simulink model "ep_10_26"  (R2023b)
settings: Solver=VariableStepAuto  StartTime=0.0  StopTime=10.0  MaxStep=0.01  RelTol=1e-3
settings Model: Creator=86186  LastModifiedBy=86186

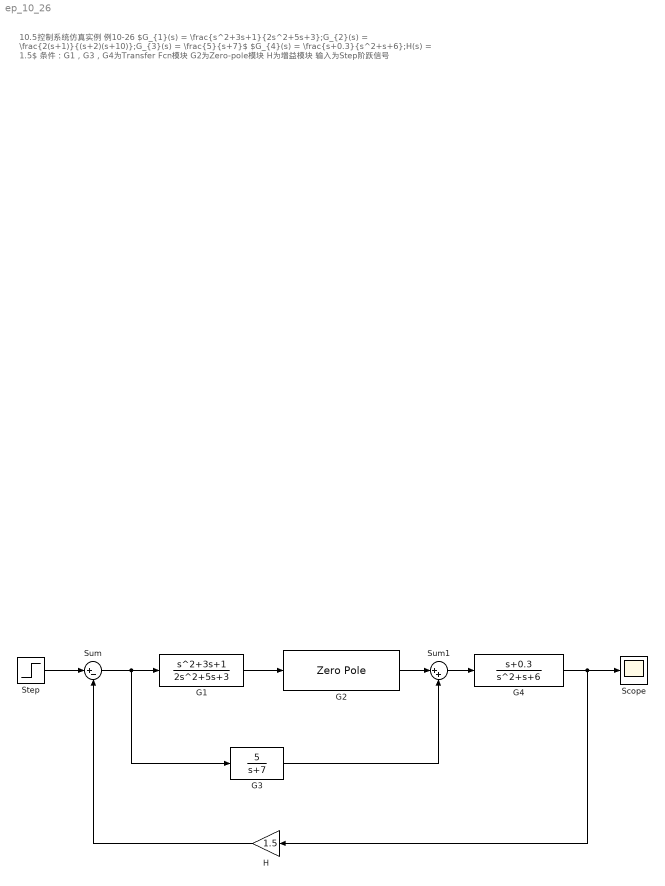
== system ep_10_26 ==
  note: 10.5控制系统仿真实例
      | 例10-26
      |
      | $G_{1}(s) = \frac{s^2+3s+1}{2s^2+5s+3};G_{2}(s) = \frac{2(s+1)}{(s+2)(s+10)};G_{3}(s) = \frac{5}{s+7}$
      | $G_{4}(s) = \frac{s+0.3}{s^2+s+6};H(s) = 1.5$
      | 条件：G1，G3，G4为Transfer Fcn模块
      | G2为Zero-pole模块
      | H为增益模块
      | 输入为Step阶跃信号
  G1 : TransferFcn  Numerator=[1 3 1]  Denominator=[2 5 3]
  G2 : ZeroPole  Zeros=[-1]  Poles=[-2 -10]  Gain=[2]
  G3 : TransferFcn  Numerator=[5]  Denominator=[1 7]
  G4 : TransferFcn  Numerator=[1 0.3]  Denominator=[1 1 6]
  H : Gain  Gain=1.5
  Scope : Scope
  Step : Step  Time=0  SampleTime=0
  Sum : Sum  Inputs=|+-
  Sum1 : Sum  Inputs=|++
  wires:
  Sum/1 -> G1/1, G3/1
  G2/1 -> Sum1/1
  G1/1 -> G2/1
  Sum1/1 -> G4/1
  G3/1 -> Sum1/2
  H/1 -> Sum/2
  G4/1 -> Scope/1, H/1
  Step/1 -> Sum/1
